simulink model "vnt_entire"  (R2018b)
settings: Solver=VariableStepAuto  StartTime=0.0  StopTime=inf  RelTol=1e-3
PreLoadFcn:
  | if exist('tl_preloadfcn','file'), tl_preloadfcn(gcs,'4.4.0.41'); end
PostLoadFcn:
  | if exist('tl_postloadfcn','file'), tl_postloadfcn(gcs,'4.4.0.41'); end
InitFcn:
  | if exist('tlds_init','file'), tlds_init(gcs); end
StartFcn:
  | if exist('tlds_start','file'), tlds_start(gcs); end
StopFcn:
  | if exist('tlds_stop','file'), tlds_stop(gcs); end
undefined symbols (not defined in the file): canChannel
libraries: canlib x29, canmsglib x27, simulink x4, pePwmGenerator x2, daqlib x1, aerolibnav x1
PreSaveFcn:
  | if exist('tl_presavefcn','file'), tl_presavefcn(gcs); end
CloseFcn:
  | if exist('tl_closefcn','file'), tl_closefcn(gcs); end
settings Model: Creator=GE72 6QF  LastModifiedBy=GE72 6QF

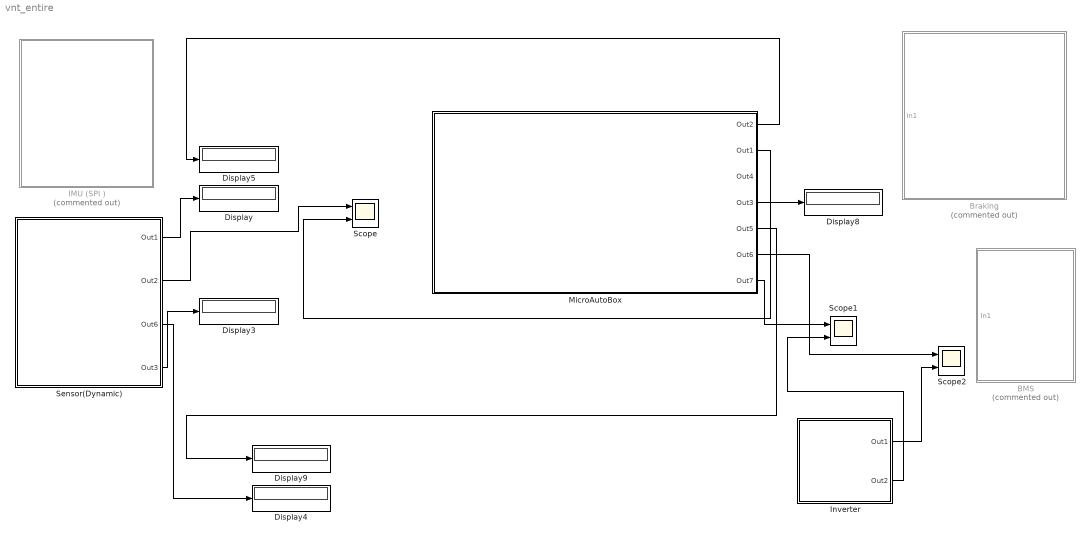
== system vnt_entire ==
  BMS : Subsystem  Commented=on
  Braking : Subsystem  Commented=on
  Display{,3..5,8..9} (6 alike) : Display
  IMU (SPI ) : Subsystem  Commented=on
  Inverter : Subsystem
  MicroAutoBox : Subsystem
  Scope : Scope  NumInputPorts=2
  Scope1 : Scope  NumInputPorts=2
  Scope2 : Scope  NumInputPorts=2
  Sensor(Dynamic) : Subsystem
  wires:
  Sensor(Dynamic)/1(Out1) -> Display/1
  Sensor(Dynamic)/3(Out6) -> Display4/1
  Inverter/2(Out2) -> Scope1/2
  MicroAutoBox/6(Out6) -> Scope2/1
  MicroAutoBox/7(Out7) -> Scope1/1
  MicroAutoBox/1(Out2) -> Display5/1
  MicroAutoBox/2(Out1) -> Scope/2
  MicroAutoBox/4(Out3) -> Display8/1
  MicroAutoBox/5(Out5) -> Display9/1
  Inverter/1(Out1) -> Scope2/2
  Sensor(Dynamic)/2(Out2) -> Scope/1
  Sensor(Dynamic)/4(Out3) -> Display3/1

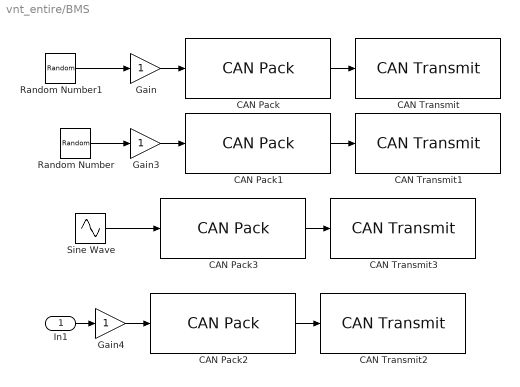
== system vnt_entire/BMS ==
  In1 : Inport
  CAN Pack : canmsglib/CAN Pack  MsgList=(none)  MsgName=CAN Msg  MsgIDType=Standard (11-bit identifier)  MsgIdentifier=100  MsgLength=8  SignalInfo=Signal1$0$8$1$1$1$0$1$0$-Inf$Inf$#  NSignals=1  StartBits=str2num('[int32(0)]')  SignalSizes=str2num('[int32(8)]')  ByteOrders=str2num('[int32(1)]')  DataTypes=str2num('[int32(1)]')  MultiplexTypes=str2num('[int32(1)]')  MultiplexValues=str2num('[double(0)]')  Factors=str2num('[double(1)]')  Offsets=str2num('[double(0)]')  Minimums=str2num('[double(-Inf)]')  Maximums=str2num('[double(Inf)]')  Remote=off  ApplyMinMax=off  BusOutput=off
      settings: SourceProductName=Simulink Real-Time  SourceProductBaseCode=XP  DataFormat=manually specified signals
  CAN Pack1 : canmsglib/CAN Pack  MsgList=(none)  MsgName=CAN Msg  MsgIDType=Standard (11-bit identifier)  MsgIdentifier=200  MsgLength=8  NSignals=0  StartBits=0  SignalSizes=0  ByteOrders=0  DataTypes=0  MultiplexTypes=0  MultiplexValues=0  Factors=0  Offsets=0  Minimums=0  Maximums=0  Remote=off  ApplyMinMax=off  BusOutput=off
      settings: SourceProductName=Simulink Real-Time  SourceProductBaseCode=XP  DataFormat=manually specified signals
  CAN Pack2 : canmsglib/CAN Pack  MsgList=(none)  MsgName=CAN Msg  MsgIDType=Standard (11-bit identifier)  MsgIdentifier=0  MsgLength=8  NSignals=0  StartBits=0  SignalSizes=0  ByteOrders=0  DataTypes=0  MultiplexTypes=0  MultiplexValues=0  Factors=0  Offsets=0  Minimums=0  Maximums=0  Remote=off  ApplyMinMax=off  BusOutput=off
      settings: SourceProductName=Simulink Real-Time  SourceProductBaseCode=XP  DataFormat=raw data
  CAN Pack3 : canmsglib/CAN Pack  MsgList=(none)  MsgName=CAN Msg  MsgIDType=Standard (11-bit identifier)  MsgIdentifier=0  MsgLength=8  NSignals=0  StartBits=0  SignalSizes=0  ByteOrders=0  DataTypes=0  MultiplexTypes=0  MultiplexValues=0  Factors=0  Offsets=0  Minimums=0  Maximums=0  Remote=off  ApplyMinMax=off  BusOutput=off
      settings: SourceProductName=Simulink Real-Time  SourceProductBaseCode=XP  DataFormat=raw data
  CAN Transmit : canlib/CAN Transmit  BlockHandle=11.0005  DeviceMenu=MathWorks Virtual 1 (Channel 1)  Device=MathWorks Virtual 1 (Channel 1)  ObjConstructor=canChannel('MathWorks', 'Virtual 1', 1)  EnablePeriodicTransmit=off  MessagePeriod=1.000
      settings: SourceProductName=Vehicle Network Toolbox  SourceProductBaseCode=VN
  CAN Transmit1 : canlib/CAN Transmit  BlockHandle=12.0005  DeviceMenu=MathWorks Virtual 1 (Channel 1)  Device=MathWorks Virtual 1 (Channel 1)  ObjConstructor=canChannel('MathWorks', 'Virtual 1', 1)  EnablePeriodicTransmit=off  MessagePeriod=1.000
      settings: SourceProductName=Vehicle Network Toolbox  SourceProductBaseCode=VN
  CAN Transmit2 : canlib/CAN Transmit  BlockHandle=13.0004  DeviceMenu=MathWorks Virtual 1 (Channel 1)  Device=MathWorks Virtual 1 (Channel 1)  ObjConstructor=canChannel('MathWorks', 'Virtual 1', 1)  EnablePeriodicTransmit=off  MessagePeriod=1.000
      settings: SourceProductName=Vehicle Network Toolbox  SourceProductBaseCode=VN
  CAN Transmit3 : canlib/CAN Transmit  BlockHandle=15.0005  DeviceMenu=MathWorks Virtual 1 (Channel 1)  Device=MathWorks Virtual 1 (Channel 1)  ObjConstructor=canChannel('MathWorks', 'Virtual 1', 1)  EnablePeriodicTransmit=off  MessagePeriod=1.000
      settings: SourceProductName=Vehicle Network Toolbox  SourceProductBaseCode=VN
  Gain : Gain
  Gain3 : Gain
  Gain4 : Gain
  Random Number : RandomNumber  SampleTime=0.1
  Random Number1 : RandomNumber  SampleTime=0.1
  Sine Wave : Sin  SampleTime=0
  wires:
  Gain4/1 -> CAN Pack2/1
  Random Number/1 -> Gain3/1
  CAN Pack3/1 -> CAN Transmit3/1
  Random Number1/1 -> Gain/1
  CAN Pack1/1 -> CAN Transmit1/1
  Gain3/1 -> CAN Pack1/1
  Gain/1 -> CAN Pack/1
  Sine Wave/1 -> CAN Pack3/1
  CAN Pack/1 -> CAN Transmit/1
  CAN Pack2/1 -> CAN Transmit2/1
  In1/1 -> Gain4/1

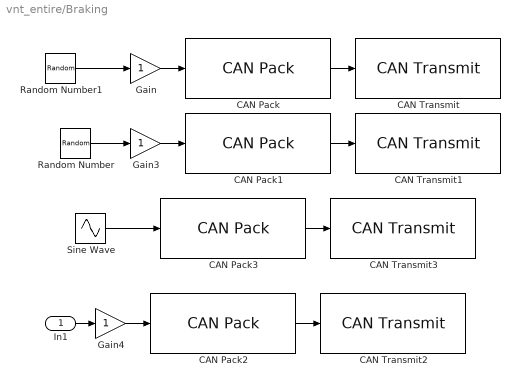
== system vnt_entire/Braking ==
  In1 : Inport
  CAN Pack : canmsglib/CAN Pack  MsgList=(none)  MsgName=CAN Msg  MsgIDType=Standard (11-bit identifier)  MsgIdentifier=100  MsgLength=8  SignalInfo=Signal1$0$8$1$1$1$0$1$0$-Inf$Inf$#  NSignals=1  StartBits=str2num('[int32(0)]')  SignalSizes=str2num('[int32(8)]')  ByteOrders=str2num('[int32(1)]')  DataTypes=str2num('[int32(1)]')  MultiplexTypes=str2num('[int32(1)]')  MultiplexValues=str2num('[double(0)]')  Factors=str2num('[double(1)]')  Offsets=str2num('[double(0)]')  Minimums=str2num('[double(-Inf)]')  Maximums=str2num('[double(Inf)]')  Remote=off  ApplyMinMax=off  BusOutput=off
      settings: SourceProductName=Simulink Real-Time  SourceProductBaseCode=XP  DataFormat=manually specified signals
  CAN Pack1 : canmsglib/CAN Pack  MsgList=(none)  MsgName=CAN Msg  MsgIDType=Standard (11-bit identifier)  MsgIdentifier=200  MsgLength=8  NSignals=0  StartBits=0  SignalSizes=0  ByteOrders=0  DataTypes=0  MultiplexTypes=0  MultiplexValues=0  Factors=0  Offsets=0  Minimums=0  Maximums=0  Remote=off  ApplyMinMax=off  BusOutput=off
      settings: SourceProductName=Simulink Real-Time  SourceProductBaseCode=XP  DataFormat=manually specified signals
  CAN Pack2 : canmsglib/CAN Pack  MsgList=(none)  MsgName=CAN Msg  MsgIDType=Standard (11-bit identifier)  MsgIdentifier=0  MsgLength=8  NSignals=0  StartBits=0  SignalSizes=0  ByteOrders=0  DataTypes=0  MultiplexTypes=0  MultiplexValues=0  Factors=0  Offsets=0  Minimums=0  Maximums=0  Remote=off  ApplyMinMax=off  BusOutput=off
      settings: SourceProductName=Simulink Real-Time  SourceProductBaseCode=XP  DataFormat=raw data
  CAN Pack3 : canmsglib/CAN Pack  MsgList=(none)  MsgName=CAN Msg  MsgIDType=Standard (11-bit identifier)  MsgIdentifier=0  MsgLength=8  NSignals=0  StartBits=0  SignalSizes=0  ByteOrders=0  DataTypes=0  MultiplexTypes=0  MultiplexValues=0  Factors=0  Offsets=0  Minimums=0  Maximums=0  Remote=off  ApplyMinMax=off  BusOutput=off
      settings: SourceProductName=Simulink Real-Time  SourceProductBaseCode=XP  DataFormat=raw data
  CAN Transmit : canlib/CAN Transmit  BlockHandle=46.0005  DeviceMenu=MathWorks Virtual 1 (Channel 1)  Device=MathWorks Virtual 1 (Channel 1)  ObjConstructor=canChannel('MathWorks', 'Virtual 1', 1)  EnablePeriodicTransmit=off  MessagePeriod=1.000
      settings: SourceProductName=Vehicle Network Toolbox  SourceProductBaseCode=VN
  CAN Transmit1 : canlib/CAN Transmit  BlockHandle=47.0005  DeviceMenu=MathWorks Virtual 1 (Channel 1)  Device=MathWorks Virtual 1 (Channel 1)  ObjConstructor=canChannel('MathWorks', 'Virtual 1', 1)  EnablePeriodicTransmit=off  MessagePeriod=1.000
      settings: SourceProductName=Vehicle Network Toolbox  SourceProductBaseCode=VN
  CAN Transmit2 : canlib/CAN Transmit  BlockHandle=48.0005  DeviceMenu=MathWorks Virtual 1 (Channel 1)  Device=MathWorks Virtual 1 (Channel 1)  ObjConstructor=canChannel('MathWorks', 'Virtual 1', 1)  EnablePeriodicTransmit=off  MessagePeriod=1.000
      settings: SourceProductName=Vehicle Network Toolbox  SourceProductBaseCode=VN
  CAN Transmit3 : canlib/CAN Transmit  BlockHandle=49.0005  DeviceMenu=MathWorks Virtual 1 (Channel 1)  Device=MathWorks Virtual 1 (Channel 1)  ObjConstructor=canChannel('MathWorks', 'Virtual 1', 1)  EnablePeriodicTransmit=off  MessagePeriod=1.000
      settings: SourceProductName=Vehicle Network Toolbox  SourceProductBaseCode=VN
  Gain : Gain
  Gain3 : Gain
  Gain4 : Gain
  Random Number : RandomNumber  SampleTime=0.1
  Random Number1 : RandomNumber  SampleTime=0.1
  Sine Wave : Sin  SampleTime=0
  wires:
  Gain4/1 -> CAN Pack2/1
  Random Number/1 -> Gain3/1
  CAN Pack3/1 -> CAN Transmit3/1
  Random Number1/1 -> Gain/1
  CAN Pack1/1 -> CAN Transmit1/1
  Gain3/1 -> CAN Pack1/1
  Gain/1 -> CAN Pack/1
  Sine Wave/1 -> CAN Pack3/1
  CAN Pack/1 -> CAN Transmit/1
  CAN Pack2/1 -> CAN Transmit2/1
  In1/1 -> Gain4/1

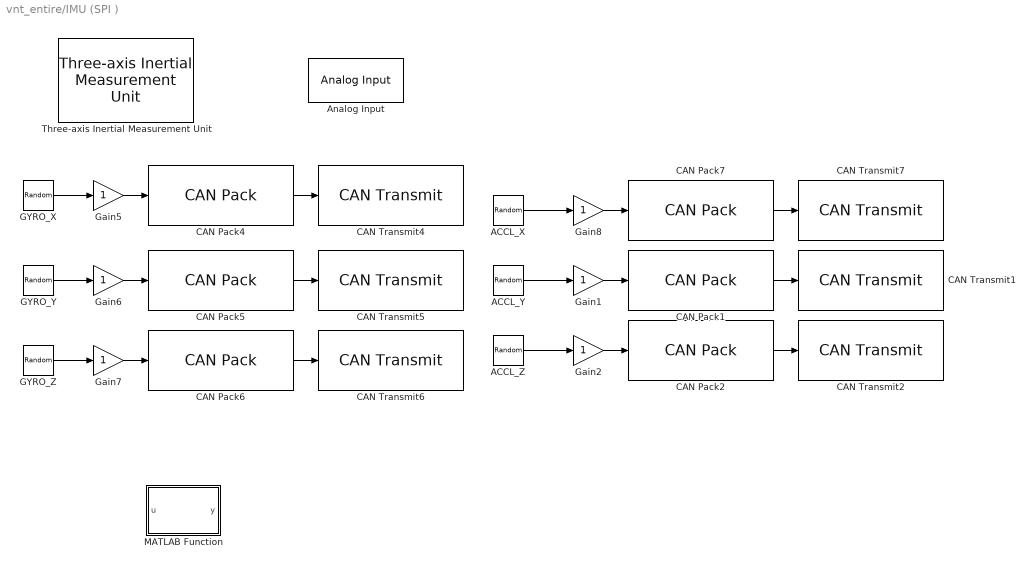
== system vnt_entire/IMU (SPI ) ==
  ACCL_X : RandomNumber  SampleTime=0.1
  ACCL_Y : RandomNumber  SampleTime=0.1
  ACCL_Z : RandomNumber  SampleTime=0.1
  Analog Input : daqlib/Analog Input  DeviceMenu=(none)  Device=(none)  NChannelsSelected=1  NPorts=1 for all channels  SampleRate=0  ActualRate=0  ScansPerTrigger=2  OutputTimestamp=off  AcqMode=0  NumFrameBuffer=100  OutputTriggertime=off
      settings: SourceProductName=Data Acquisition Toolbox  SourceProductBaseCode=DA
  CAN Pack{1..2,5..7} (5 alike) : canmsglib/CAN Pack  MsgList=(none)  MsgName=CAN Msg  MsgIDType=Standard (11-bit identifier)  MsgIdentifier=0  MsgLength=8  NSignals=0  StartBits=0  SignalSizes=0  ByteOrders=0  DataTypes=0  MultiplexTypes=0  MultiplexValues=0  Factors=0  Offsets=0  Minimums=0  Maximums=0  Remote=off  ApplyMinMax=off  BusOutput=off
      settings: SourceProductName=Simulink Real-Time  SourceProductBaseCode=XP  DataFormat=raw data
  CAN Pack4 : canmsglib/CAN Pack  MsgList=(none)  MsgName=CAN Msg  MsgIDType=Standard (11-bit identifier)  MsgIdentifier=150  MsgLength=8  SignalInfo=Signal1$0$8$1$1$1$0$1$0$-Inf$Inf$#  NSignals=1  StartBits=str2num('[int32(0)]')  SignalSizes=str2num('[int32(8)]')  ByteOrders=str2num('[int32(1)]')  DataTypes=str2num('[int32(1)]')  MultiplexTypes=str2num('[int32(1)]')  MultiplexValues=str2num('[double(0)]')  Factors=str2num('[double(1)]')  Offsets=str2num('[double(0)]')  Minimums=str2num('[double(-Inf)]')  Maximums=str2num('[double(Inf)]')  Remote=off  ApplyMinMax=off  BusOutput=off
      settings: SourceProductName=Simulink Real-Time  SourceProductBaseCode=XP  DataFormat=manually specified signals
  CAN Transmit1 : canlib/CAN Transmit  BlockHandle=84.001  DeviceMenu=MathWorks Virtual 1 (Channel 1)  Device=MathWorks Virtual 1 (Channel 1)  ObjConstructor=canChannel('MathWorks', 'Virtual 1', 1)  EnablePeriodicTransmit=off  MessagePeriod=1.000
      settings: SourceProductName=Vehicle Network Toolbox  SourceProductBaseCode=VN
  CAN Transmit2 : canlib/CAN Transmit  BlockHandle=85.0006  DeviceMenu=MathWorks Virtual 1 (Channel 1)  Device=MathWorks Virtual 1 (Channel 1)  ObjConstructor=canChannel('MathWorks', 'Virtual 1', 1)  EnablePeriodicTransmit=off  MessagePeriod=1.000
      settings: SourceProductName=Vehicle Network Toolbox  SourceProductBaseCode=VN
  CAN Transmit4 : canlib/CAN Transmit  BlockHandle=86.0006  DeviceMenu=MathWorks Virtual 1 (Channel 1)  Device=MathWorks Virtual 1 (Channel 1)  ObjConstructor=canChannel('MathWorks', 'Virtual 1', 1)  EnablePeriodicTransmit=off  MessagePeriod=1.000
      settings: SourceProductName=Vehicle Network Toolbox  SourceProductBaseCode=VN
  CAN Transmit5 : canlib/CAN Transmit  BlockHandle=87.0007  DeviceMenu=MathWorks Virtual 1 (Channel 1)  Device=MathWorks Virtual 1 (Channel 1)  ObjConstructor=canChannel('MathWorks', 'Virtual 1', 1)  EnablePeriodicTransmit=off  MessagePeriod=1.000
      settings: SourceProductName=Vehicle Network Toolbox  SourceProductBaseCode=VN
  CAN Transmit6 : canlib/CAN Transmit  BlockHandle=88.0007  DeviceMenu=MathWorks Virtual 1 (Channel 1)  Device=MathWorks Virtual 1 (Channel 1)  ObjConstructor=canChannel('MathWorks', 'Virtual 1', 1)  EnablePeriodicTransmit=off  MessagePeriod=1.000
      settings: SourceProductName=Vehicle Network Toolbox  SourceProductBaseCode=VN
  CAN Transmit7 : canlib/CAN Transmit  BlockHandle=89.0009  DeviceMenu=MathWorks Virtual 1 (Channel 1)  Device=MathWorks Virtual 1 (Channel 1)  ObjConstructor=canChannel('MathWorks', 'Virtual 1', 1)  EnablePeriodicTransmit=off  MessagePeriod=1.000
      settings: SourceProductName=Vehicle Network Toolbox  SourceProductBaseCode=VN
  GYRO_X : RandomNumber  SampleTime=0.1
  GYRO_Y : RandomNumber  SampleTime=0.1
  GYRO_Z : RandomNumber  SampleTime=0.1
  Gain{1..2,5..8} (6 alike) : Gain
  MATLAB Function : MATLAB Function  TreatAsAtomicUnit=on
  Three-axis Inertial Measurement Unit : aerolibnav/Three-axis Inertial Measurement Unit  units=Metric (MKS)  imu=[0 0 0]  i_Ts=0  dtype_a=on  w_a=190  z_a=0.707  a_sf_cc=[1 0 0; 0 1 0; 0 0 1]  a_bias=[0 0 0]  a_sat="[-inf  -inf  -inf  inf inf inf]"  dtype_g=on  w_g=190  z_g=0.707  g_sf_cc=[1 0 0; 0 1 0; 0 0 1]  g_bias=[0 0 0]  g_sens=[0 0 0]  g_sat="[-inf  -inf  -inf  inf inf inf]"  i_rand=on  i_seeds=[23093 23094 23095 23096 23097 23098]  i_pow=[0.001 0.001 0.001 0.0001 0.0001 0.0001]
  wires:
  Gain7/1 -> CAN Pack6/1
  CAN Pack5/1 -> CAN Transmit5/1
  Gain5/1 -> CAN Pack4/1
  CAN Pack4/1 -> CAN Transmit4/1
  Gain6/1 -> CAN Pack5/1
  Gain8/1 -> CAN Pack7/1
  CAN Pack7/1 -> CAN Transmit7/1
  CAN Pack6/1 -> CAN Transmit6/1
  ACCL_X/1 -> Gain8/1
  GYRO_X/1 -> Gain5/1
  GYRO_Z/1 -> Gain7/1
  GYRO_Y/1 -> Gain6/1
  Gain1/1 -> CAN Pack1/1
  CAN Pack1/1 -> CAN Transmit1/1
  ACCL_Y/1 -> Gain1/1
  Gain2/1 -> CAN Pack2/1
  CAN Pack2/1 -> CAN Transmit2/1
  ACCL_Z/1 -> Gain2/1

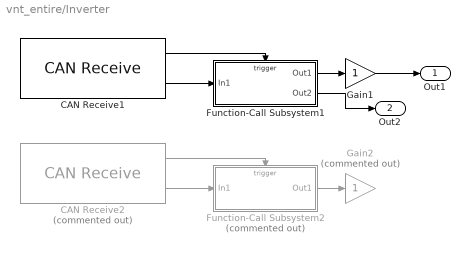
== system vnt_entire/Inverter ==
  CAN Receive1 : canlib/CAN Receive  BlockHandle=117.0006  DeviceMenu=MathWorks Virtual 1 (Channel 2)  Device=MathWorks Virtual 1 (Channel 2)  ObjConstructor=canChannel('MathWorks', 'Virtual 1', 2)  EnableStandardIDsFilter=off  StandardIDs=90  EnableExtendedIDsFilter=off  ExtendedIDs=0  SampleTime=0.01  MsgsPerTimestep=all  StdIDsCombo=Allow only  ExtIDsCombo=Allow all  InternalFilterUpdateStatus=on  BusOutput=off
      settings: SourceProductName=Vehicle Network Toolbox  SourceProductBaseCode=VN
  CAN Receive2 : canlib/CAN Receive  Commented=on  BlockHandle=118.0007  DeviceMenu=MathWorks Virtual 1 (Channel 2)  Device=MathWorks Virtual 1 (Channel 2)  ObjConstructor=canChannel('MathWorks', 'Virtual 1', 2)  EnableStandardIDsFilter=off  StandardIDs=90  EnableExtendedIDsFilter=off  ExtendedIDs=0  SampleTime=0.01  MsgsPerTimestep=all  StdIDsCombo=Allow only  ExtIDsCombo=Allow all  InternalFilterUpdateStatus=on  BusOutput=off
      settings: SourceProductName=Vehicle Network Toolbox  SourceProductBaseCode=VN
  Function-Call Subsystem1 : Subsystem  TreatAsAtomicUnit=on
  Function-Call Subsystem2 : Subsystem  Commented=on  TreatAsAtomicUnit=on
  Gain1 : Gain
  Gain2 : Gain  Commented=on
  Out1 : Outport
  Out2 : Outport  Port=2
  wires:
  Function-Call Subsystem2/1(Out1) -> Gain2/1
  CAN Receive1/1 -> Function-Call Subsystem1/Trigger
  Function-Call Subsystem1/1(Out1) -> Gain1/1
  CAN Receive2/2 -> Function-Call Subsystem2/1(In1)
  CAN Receive2/1 -> Function-Call Subsystem2/Trigger
  CAN Receive1/2 -> Function-Call Subsystem1/1(In1)
  Gain1/1 -> Out1/1
  Function-Call Subsystem1/2(Out2) -> Out2/1

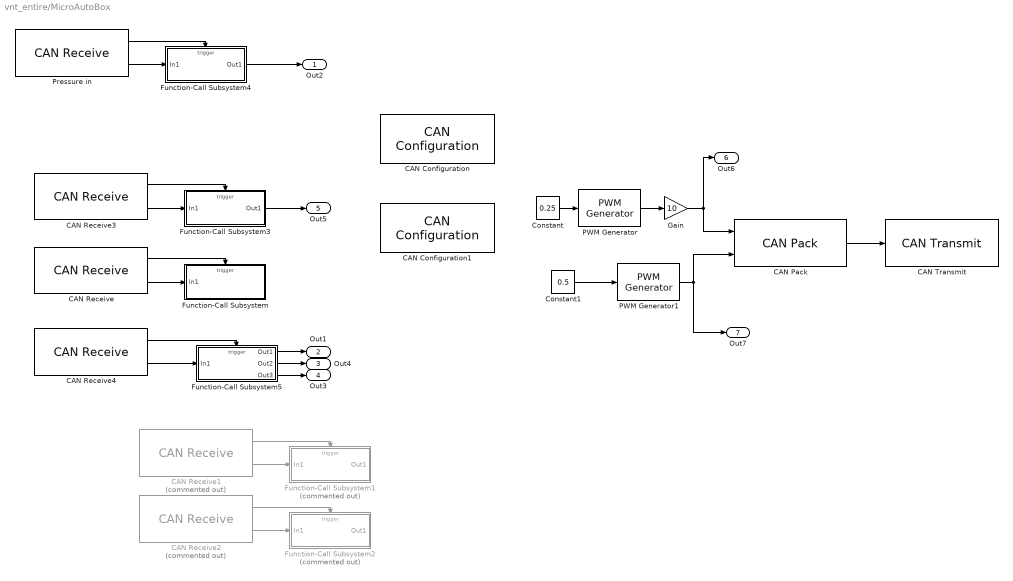
== system vnt_entire/MicroAutoBox ==
  CAN Configuration : canlib/CAN Configuration  BlockHandle=148.0005  DeviceMenu=MathWorks Virtual 1 (Channel 1)  Device=MathWorks Virtual 1 (Channel 1)  ObjConstructor=canChannel('MathWorks', 'Virtual 1', 1)  BusSpeed=500000  EnableBitParameters=off  AckMode=Normal
      settings: SourceProductName=Vehicle Network Toolbox  SourceProductBaseCode=VN
  CAN Configuration1 : canlib/CAN Configuration  BlockHandle=149.0005  DeviceMenu=MathWorks Virtual 1 (Channel 2)  Device=MathWorks Virtual 1 (Channel 2)  ObjConstructor=canChannel('MathWorks', 'Virtual 1', 2)  BusSpeed=500000  EnableBitParameters=off  AckMode=Normal
      settings: SourceProductName=Vehicle Network Toolbox  SourceProductBaseCode=VN
  CAN Pack : canmsglib/CAN Pack  MsgList=(none)  MsgName=CAN Msg  MsgIDType=Standard (11-bit identifier)  MsgIdentifier=90  MsgLength=8  SignalInfo=Signal1$0$32$1$3$1$0$1$0$-Inf$Inf$#Signal2$32$32$1$3$1$0$1$0$-Inf$Inf$#  NSignals=2  StartBits=str2num('[int32(0);int32(32)]')  SignalSizes=str2num('[int32(32);int32(32)]')  ByteOrders=str2num('[int32(1);int32(1)]')  DataTypes=str2num('[int32(3);int32(3)]')  MultiplexTypes=str2num('[int32(1);int32(1)]')  MultiplexValues=str2num('[double(0);double(0)]')  Factors=str2num('[double(1);double(1)]')  Offsets=str2num('[double(0);double(0)]')  Minimums=str2num('[double(-Inf);double(-Inf)]')  Maximums=str2num('[double(Inf);double(Inf)]')  Remote=off  ApplyMinMax=off  BusOutput=off
      settings: SourceProductName=Simulink Real-Time  SourceProductBaseCode=XP  DataFormat=manually specified signals
  CAN Receive : canlib/CAN Receive  BlockHandle=151.0006  DeviceMenu=MathWorks Virtual 1 (Channel 1)  Device=MathWorks Virtual 1 (Channel 1)  ObjConstructor=canChannel('MathWorks', 'Virtual 1', 1)  EnableStandardIDsFilter=off  StandardIDs=220  EnableExtendedIDsFilter=off  ExtendedIDs=0  SampleTime=0.01  MsgsPerTimestep=all  StdIDsCombo=Allow only  ExtIDsCombo=Allow all  InternalFilterUpdateStatus=on  BusOutput=off
      settings: SourceProductName=Vehicle Network Toolbox  SourceProductBaseCode=VN
  CAN Receive1 : canlib/CAN Receive  Commented=on  BlockHandle=152.0007  DeviceMenu=MathWorks Virtual 1 (Channel 1)  Device=MathWorks Virtual 1 (Channel 1)  ObjConstructor=canChannel('MathWorks', 'Virtual 1', 1)  EnableStandardIDsFilter=off  StandardIDs=0  EnableExtendedIDsFilter=off  ExtendedIDs=0  SampleTime=0.01  MsgsPerTimestep=all  StdIDsCombo=Allow all  ExtIDsCombo=Allow all  InternalFilterUpdateStatus=off  BusOutput=off
      settings: SourceProductName=Vehicle Network Toolbox  SourceProductBaseCode=VN
  CAN Receive2 : canlib/CAN Receive  Commented=on  BlockHandle=153.0006  DeviceMenu=MathWorks Virtual 1 (Channel 1)  Device=MathWorks Virtual 1 (Channel 1)  ObjConstructor=canChannel('MathWorks', 'Virtual 1', 1)  EnableStandardIDsFilter=off  StandardIDs=0  EnableExtendedIDsFilter=off  ExtendedIDs=0  SampleTime=0.01  MsgsPerTimestep=all  StdIDsCombo=Allow all  ExtIDsCombo=Allow all  InternalFilterUpdateStatus=off  BusOutput=off
      settings: SourceProductName=Vehicle Network Toolbox  SourceProductBaseCode=VN
  CAN Receive3 : canlib/CAN Receive  BlockHandle=154.0013  DeviceMenu=MathWorks Virtual 1 (Channel 2)  Device=MathWorks Virtual 1 (Channel 2)  ObjConstructor=canChannel('MathWorks', 'Virtual 1', 2)  EnableStandardIDsFilter=off  StandardIDs=230  EnableExtendedIDsFilter=off  ExtendedIDs=0  SampleTime=0.01  MsgsPerTimestep=all  StdIDsCombo=Allow only  ExtIDsCombo=Allow all  InternalFilterUpdateStatus=on  BusOutput=off
      settings: SourceProductName=Vehicle Network Toolbox  SourceProductBaseCode=VN
  CAN Receive4 : canlib/CAN Receive  BlockHandle=155.0007  DeviceMenu=MathWorks Virtual 1 (Channel 1)  Device=MathWorks Virtual 1 (Channel 1)  ObjConstructor=canChannel('MathWorks', 'Virtual 1', 1)  EnableStandardIDsFilter=off  StandardIDs=210  EnableExtendedIDsFilter=off  ExtendedIDs=0  SampleTime=0.01  MsgsPerTimestep=all  StdIDsCombo=Allow only  ExtIDsCombo=Allow all  InternalFilterUpdateStatus=on  BusOutput=off
      settings: SourceProductName=Vehicle Network Toolbox  SourceProductBaseCode=VN
  CAN Transmit : canlib/CAN Transmit  BlockHandle=156.0006  DeviceMenu=MathWorks Virtual 1 (Channel 2)  Device=MathWorks Virtual 1 (Channel 2)  ObjConstructor=canChannel('MathWorks', 'Virtual 1', 2)  EnablePeriodicTransmit=off  MessagePeriod=1.000
      settings: SourceProductName=Vehicle Network Toolbox  SourceProductBaseCode=VN
  Constant : Constant  Value=0.25
  Constant1 : Constant  Value=0.5
  Function-Call Subsystem : Subsystem  TreatAsAtomicUnit=on
  Function-Call Subsystem1 : Subsystem  Commented=on  TreatAsAtomicUnit=on
  Function-Call Subsystem2 : Subsystem  Commented=on  TreatAsAtomicUnit=on
  Function-Call Subsystem3 : Subsystem  TreatAsAtomicUnit=on
  Function-Call Subsystem4 : Subsystem  TreatAsAtomicUnit=on
  Function-Call Subsystem5 : Subsystem  TreatAsAtomicUnit=on
  Gain : Gain  Gain=10
  PWM Generator : pePwmGenerator/PWM Generator  CarrCount=Up  Tper=4  Ts=0.05
  PWM Generator1 : pePwmGenerator/PWM Generator  CarrCount=Up  Tper=4  Ts=0.05
  Pressure in : canlib/CAN Receive  BlockHandle=265.0013  DeviceMenu=MathWorks Virtual 1 (Channel 1)  Device=MathWorks Virtual 1 (Channel 1)  ObjConstructor=canChannel('MathWorks', 'Virtual 1', 1)  EnableStandardIDsFilter=off  StandardIDs=300  EnableExtendedIDsFilter=off  ExtendedIDs=0  SampleTime=0.01  MsgsPerTimestep=all  StdIDsCombo=Allow only  ExtIDsCombo=Allow all  InternalFilterUpdateStatus=on  BusOutput=off
      settings: SourceProductName=Vehicle Network Toolbox  SourceProductBaseCode=VN
  Out2 : Outport
  Out1 : Outport  Port=2
  Out4 : Outport  Port=3
  Out3 : Outport  Port=4
  Out5 : Outport  Port=5
  Out6 : Outport  Port=6
  Out7 : Outport  Port=7
  wires:
  CAN Receive/2 -> Function-Call Subsystem/1(In1)
  CAN Receive1/1 -> Function-Call Subsystem1/Trigger
  CAN Receive1/2 -> Function-Call Subsystem1/1(In1)
  CAN Receive2/1 -> Function-Call Subsystem2/Trigger
  CAN Receive2/2 -> Function-Call Subsystem2/1(In1)
  CAN Receive3/2 -> Function-Call Subsystem3/1(In1)
  Constant/1 -> PWM Generator/1
  CAN Pack/1 -> CAN Transmit/1
  PWM Generator/1 -> Gain/1
  Constant1/1 -> PWM Generator1/1
  Pressure in/2 -> Function-Call Subsystem4/1(In1)
  Function-Call Subsystem4/1(Out1) -> Out2/1
  CAN Receive4/2 -> Function-Call Subsystem5/1(In1)
  Function-Call Subsystem5/1(Out1) -> Out1/1
  Function-Call Subsystem5/2(Out2) -> Out4/1
  Function-Call Subsystem3/1(Out1) -> Out5/1
  Function-Call Subsystem5/3(Out3) -> Out3/1
  PWM Generator1/1 -> Out7/1, CAN Pack/2
  CAN Receive4/1 -> Function-Call Subsystem5/Trigger
  CAN Receive/1 -> Function-Call Subsystem/Trigger
  CAN Receive3/1 -> Function-Call Subsystem3/Trigger
  Pressure in/1 -> Function-Call Subsystem4/Trigger
  Gain/1 -> CAN Pack/1, Out6/1

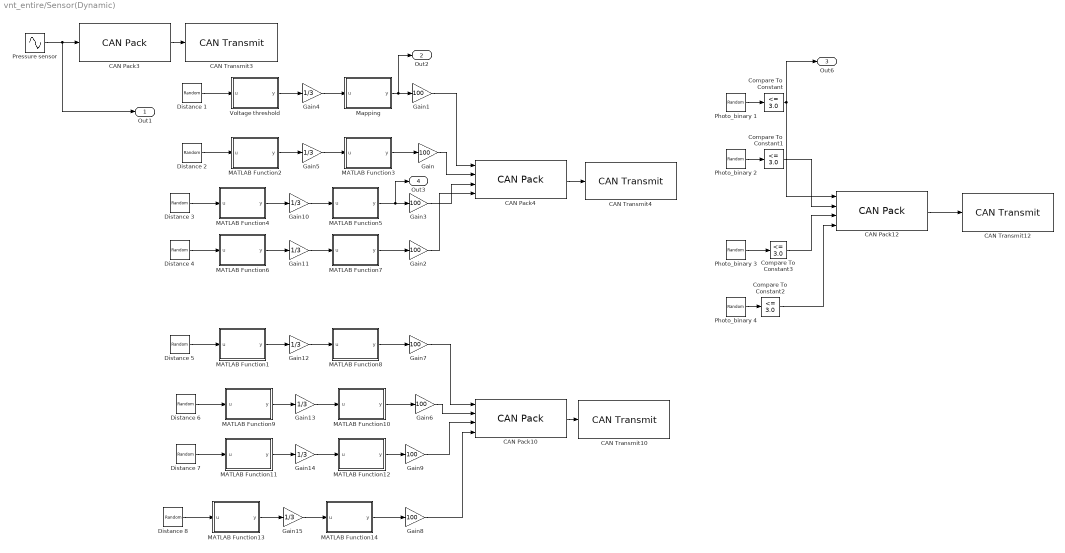
== system vnt_entire/Sensor(Dynamic) ==
  CAN Pack10 : canmsglib/CAN Pack  MsgList=(none)  MsgName=CAN Msg  MsgIDType=Standard (11-bit identifier)  MsgIdentifier=220  MsgLength=8  SignalInfo=Signal1$0$16$1$2$1$0$1$0$-Inf$Inf$#Signal2$16$16$1$2$1$0$1$0$-Inf$Inf$#Signal3$32$16$1$2$1$0$1$0$-Inf$Inf$#Signal4$48$16$1$2$1$0$1$0$-Inf$Inf$#  NSignals=4  StartBits=str2num('[int32(0);int32(16);int32(32);int32(48)]')  SignalSizes=str2num('[int32(16);int32(16);int32(16);int32(16)]')  ByteOrders=str2num('[int32(1);int32(1);int32(1);int32(1)]')  DataTypes=str2num('[int32(2);int32(2);int32(2);int32(2)]')  MultiplexTypes=str2num('[int32(1);int32(1);int32(1);int32(1)]')  MultiplexValues=str2num('[double(0);double(0);double(0);double(0)]')  Factors=str2num('[double(1);double(1);double(1);double(1)]')  Offsets=str2num('[double(0);double(0);double(0);double(0)]')  Minimums=str2num('[double(-Inf);double(-Inf);double(-Inf);double(-Inf)]')  Maximums=str2num('[double(Inf);double(Inf);double(Inf);double(Inf)]')  Remote=off  ApplyMinMax=off  BusOutput=off
      settings: SourceProductName=Simulink Real-Time  SourceProductBaseCode=XP  DataFormat=manually specified signals
  CAN Pack12 : canmsglib/CAN Pack  MsgList=(none)  MsgName=CAN Msg  MsgIDType=Standard (11-bit identifier)  MsgIdentifier=230  MsgLength=8  SignalInfo=Signal1$0$2$1$2$1$0$1$0$-Inf$Inf$#Signal2$2$2$1$2$1$0$1$0$-Inf$Inf$#Signal3$4$2$1$2$1$0$1$0$-Inf$Inf$#Signal4$6$2$1$2$1$0$1$0$-Inf$Inf$#  NSignals=4  StartBits=str2num('[int32(0);int32(2);int32(4);int32(6)]')  SignalSizes=str2num('[int32(2);int32(2);int32(2);int32(2)]')  ByteOrders=str2num('[int32(1);int32(1);int32(1);int32(1)]')  DataTypes=str2num('[int32(2);int32(2);int32(2);int32(2)]')  MultiplexTypes=str2num('[int32(1);int32(1);int32(1);int32(1)]')  MultiplexValues=str2num('[double(0);double(0);double(0);double(0)]')  Factors=str2num('[double(1);double(1);double(1);double(1)]')  Offsets=str2num('[double(0);double(0);double(0);double(0)]')  Minimums=str2num('[double(-Inf);double(-Inf);double(-Inf);double(-Inf)]')  Maximums=str2num('[double(Inf);double(Inf);double(Inf);double(Inf)]')  Remote=off  ApplyMinMax=off  BusOutput=off
      settings: SourceProductName=Simulink Real-Time  SourceProductBaseCode=XP  DataFormat=manually specified signals
  CAN Pack3 : canmsglib/CAN Pack  MsgList=(none)  MsgName=CAN Msg  MsgIDType=Standard (11-bit identifier)  MsgIdentifier=300  MsgLength=8  SignalInfo=Signal1$0$64$1$4$1$0$1$0$-Inf$Inf$#  NSignals=1  StartBits=str2num('[int32(0)]')  SignalSizes=str2num('[int32(64)]')  ByteOrders=str2num('[int32(1)]')  DataTypes=str2num('[int32(4)]')  MultiplexTypes=str2num('[int32(1)]')  MultiplexValues=str2num('[double(0)]')  Factors=str2num('[double(1)]')  Offsets=str2num('[double(0)]')  Minimums=str2num('[double(-Inf)]')  Maximums=str2num('[double(Inf)]')  Remote=off  ApplyMinMax=off  BusOutput=off
      settings: SourceProductName=Simulink Real-Time  SourceProductBaseCode=XP  DataFormat=manually specified signals
  CAN Pack4 : canmsglib/CAN Pack  MsgList=(none)  MsgName=CAN Msg  MsgIDType=Standard (11-bit identifier)  MsgIdentifier=210  MsgLength=8  SignalInfo=Signal1$0$16$1$2$1$0$1$0$-Inf$Inf$#Signal2$16$16$1$2$1$0$1$0$-Inf$Inf$#Signal3$32$16$1$2$1$0$1$0$-Inf$Inf$#Signal4$48$16$1$2$1$0$1$0$-Inf$Inf$#  NSignals=4  StartBits=str2num('[int32(0);int32(16);int32(32);int32(48)]')  SignalSizes=str2num('[int32(16);int32(16);int32(16);int32(16)]')  ByteOrders=str2num('[int32(1);int32(1);int32(1);int32(1)]')  DataTypes=str2num('[int32(2);int32(2);int32(2);int32(2)]')  MultiplexTypes=str2num('[int32(1);int32(1);int32(1);int32(1)]')  MultiplexValues=str2num('[double(0);double(0);double(0);double(0)]')  Factors=str2num('[double(1);double(1);double(1);double(1)]')  Offsets=str2num('[double(0);double(0);double(0);double(0)]')  Minimums=str2num('[double(-Inf);double(-Inf);double(-Inf);double(-Inf)]')  Maximums=str2num('[double(Inf);double(Inf);double(Inf);double(Inf)]')  Remote=off  ApplyMinMax=off  BusOutput=off
      settings: SourceProductName=Simulink Real-Time  SourceProductBaseCode=XP  DataFormat=manually specified signals
  CAN Transmit10 : canlib/CAN Transmit  BlockHandle=320.0005  DeviceMenu=MathWorks Virtual 1 (Channel 1)  Device=MathWorks Virtual 1 (Channel 1)  ObjConstructor=canChannel('MathWorks', 'Virtual 1', 1)  EnablePeriodicTransmit=off  MessagePeriod=1.000
      settings: SourceProductName=Vehicle Network Toolbox  SourceProductBaseCode=VN
  CAN Transmit12 : canlib/CAN Transmit  BlockHandle=321.0005  DeviceMenu=MathWorks Virtual 1 (Channel 1)  Device=MathWorks Virtual 1 (Channel 1)  ObjConstructor=canChannel('MathWorks', 'Virtual 1', 1)  EnablePeriodicTransmit=off  MessagePeriod=1.000
      settings: SourceProductName=Vehicle Network Toolbox  SourceProductBaseCode=VN
  CAN Transmit3 : canlib/CAN Transmit  BlockHandle=322.0005  DeviceMenu=MathWorks Virtual 1 (Channel 2)  Device=MathWorks Virtual 1 (Channel 2)  ObjConstructor=canChannel('MathWorks', 'Virtual 1', 2)  EnablePeriodicTransmit=off  MessagePeriod=1.000
      settings: SourceProductName=Vehicle Network Toolbox  SourceProductBaseCode=VN
  CAN Transmit4 : canlib/CAN Transmit  BlockHandle=323.0005  DeviceMenu=MathWorks Virtual 1 (Channel 1)  Device=MathWorks Virtual 1 (Channel 1)  ObjConstructor=canChannel('MathWorks', 'Virtual 1', 1)  EnablePeriodicTransmit=off  MessagePeriod=1.000
      settings: SourceProductName=Vehicle Network Toolbox  SourceProductBaseCode=VN
  Compare To Constant{,1..3} (4 alike) : simulink/Logic and Bit Operations/Compare To Constant  relop=<=  const=3.0  OutDataTypeStr=boolean
  Distance {1..8} (8 alike) : RandomNumber  Mean=5  Variance=5  SampleTime=0.1
  Gain{,1..3,6..9} (8 alike) : Gain  Gain=100
  Gain{4..5,10..15} (8 alike) : Gain  Gain=1/3
  MATLAB Function1 : MATLAB Function  TreatAsAtomicUnit=on
  MATLAB Function10 : MATLAB Function  TreatAsAtomicUnit=on
  MATLAB Function11 : MATLAB Function  TreatAsAtomicUnit=on
  MATLAB Function12 : MATLAB Function  TreatAsAtomicUnit=on
  MATLAB Function13 : MATLAB Function  TreatAsAtomicUnit=on
  MATLAB Function14 : MATLAB Function  TreatAsAtomicUnit=on
  MATLAB Function2 : MATLAB Function  TreatAsAtomicUnit=on
  MATLAB Function3 : MATLAB Function  TreatAsAtomicUnit=on
  MATLAB Function4 : MATLAB Function  TreatAsAtomicUnit=on
  MATLAB Function5 : MATLAB Function  TreatAsAtomicUnit=on
  MATLAB Function6 : MATLAB Function  TreatAsAtomicUnit=on
  MATLAB Function7 : MATLAB Function  TreatAsAtomicUnit=on
  MATLAB Function8 : MATLAB Function  TreatAsAtomicUnit=on
  MATLAB Function9 : MATLAB Function  TreatAsAtomicUnit=on
  "Mapping " : MATLAB Function  TreatAsAtomicUnit=on
  Photo_binary {1..4} (4 alike) : RandomNumber  Mean=3  SampleTime=0.1
  Pressure sensor : Sin  Amplitude=800  Bias=101300  SampleTime=0.001
  "Voltage threshold " : MATLAB Function  TreatAsAtomicUnit=on
  Out1 : Outport
  Out2 : Outport  Port=2
  Out6 : Outport  Port=3
  Out3 : Outport  Port=4
  wires:
  CAN Pack3/1 -> CAN Transmit3/1
  Gain3/1 -> CAN Pack4/3
  Gain/1 -> CAN Pack4/2
  Pressure sensor/1 -> Out1/1, CAN Pack3/1
  Gain1/1 -> CAN Pack4/1
  CAN Pack4/1 -> CAN Transmit4/1
  Gain2/1 -> CAN Pack4/4
  Photo_binary 1/1 -> Compare To Constant/1
  Gain6/1 -> CAN Pack10/2
  Gain9/1 -> CAN Pack10/3
  Compare To Constant3/1 -> CAN Pack12/3
  Gain7/1 -> CAN Pack10/1
  CAN Pack10/1 -> CAN Transmit10/1
  Photo_binary 3/1 -> Compare To Constant3/1
  Gain8/1 -> CAN Pack10/4
  CAN Pack12/1 -> CAN Transmit12/1
  Photo_binary 2/1 -> Compare To Constant1/1
  Compare To Constant1/1 -> CAN Pack12/2
  Photo_binary 4/1 -> Compare To Constant2/1
  Compare To Constant/1 -> CAN Pack12/1, Out6/1
  Compare To Constant2/1 -> CAN Pack12/4
  Distance 1/1 -> "Voltage threshold "/1(u)
  "Voltage threshold "/1(y) -> Gain4/1
  Gain4/1 -> "Mapping "/1(u)
  "Mapping "/1(y) -> Out2/1, Gain1/1
  Gain5/1 -> MATLAB Function3/1(u)
  Distance 2/1 -> MATLAB Function2/1(u)
  MATLAB Function3/1(y) -> Gain/1
  MATLAB Function2/1(y) -> Gain5/1
  MATLAB Function4/1(y) -> Gain10/1
  Gain10/1 -> MATLAB Function5/1(u)
  Distance 3/1 -> MATLAB Function4/1(u)
  MATLAB Function5/1(y) -> Out3/1, Gain3/1
  MATLAB Function6/1(y) -> Gain11/1
  Gain11/1 -> MATLAB Function7/1(u)
  Distance 4/1 -> MATLAB Function6/1(u)
  MATLAB Function7/1(y) -> Gain2/1
  Distance 5/1 -> MATLAB Function1/1(u)
  Gain12/1 -> MATLAB Function8/1(u)
  MATLAB Function1/1(y) -> Gain12/1
  MATLAB Function8/1(y) -> Gain7/1
  MATLAB Function10/1(y) -> Gain6/1
  Distance 6/1 -> MATLAB Function9/1(u)
  Gain13/1 -> MATLAB Function10/1(u)
  MATLAB Function9/1(y) -> Gain13/1
  MATLAB Function12/1(y) -> Gain9/1
  Distance 7/1 -> MATLAB Function11/1(u)
  Gain14/1 -> MATLAB Function12/1(u)
  MATLAB Function11/1(y) -> Gain14/1
  Distance 8/1 -> MATLAB Function13/1(u)
  Gain15/1 -> MATLAB Function14/1(u)
  MATLAB Function13/1(y) -> Gain15/1
  MATLAB Function14/1(y) -> Gain8/1

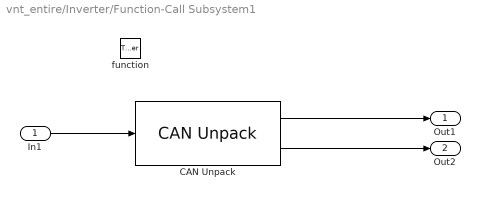
== system vnt_entire/Inverter/Function-Call Subsystem1 ==
  In1 : Inport
  function : TriggerPort  TriggerType=function-call  VariantControl=Variant
  CAN Unpack : canmsglib/CAN Unpack  MsgList=(none)  MsgName=CAN Msg  MsgIDType=Standard (11-bit identifier)  MsgIdentifier=90  MsgLength=8  SignalInfo=Signal1$0$32$1$3$1$0$1$0$-Inf$Inf$#Signal2$32$32$1$3$1$0$1$0$-Inf$Inf$#  NSignals=2  IDPort=off  TimestampPort=off  ErrorPort=off  RemotePort=off  LengthPort=off  StatusPort=off  StartBits=str2num('[int32(0);int32(32)]')  SignalSizes=str2num('[int32(32);int32(32)]')  ByteOrders=str2num('[int32(1);int32(1)]')  DataTypes=str2num('[int32(3);int32(3)]')  MultiplexTypes=str2num('[int32(1);int32(1)]')  MultiplexValues=str2num('[double(0);double(0)]')  Factors=str2num('[double(1);double(1)]')  Offsets=str2num('[double(0);double(0)]')  Minimums=str2num('[double(-Inf);double(-Inf)]')  Maximums=str2num('[double(Inf);double(Inf)]')  ApplyMinMax=off
      settings: SourceProductName=Simulink Real-Time  SourceProductBaseCode=XP
  Out1 : Outport
  Out2 : Outport  Port=2
  wires:
  In1/1 -> CAN Unpack/1
  CAN Unpack/1 -> Out1/1
  CAN Unpack/2 -> Out2/1

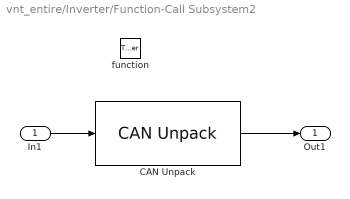
== system vnt_entire/Inverter/Function-Call Subsystem2 ==
  In1 : Inport
  function : TriggerPort  TriggerType=function-call  VariantControl=Variant
  CAN Unpack : canmsglib/CAN Unpack  MsgList=(none)  MsgName=CAN Msg  MsgIDType=Standard (11-bit identifier)  MsgIdentifier=90  MsgLength=8  SignalInfo=Signal1$0$8$1$1$1$0$1$0$-Inf$Inf$#  NSignals=1  IDPort=off  TimestampPort=off  ErrorPort=off  RemotePort=off  LengthPort=off  StatusPort=off  StartBits=str2num('[int32(0)]')  SignalSizes=str2num('[int32(8)]')  ByteOrders=str2num('[int32(1)]')  DataTypes=str2num('[int32(1)]')  MultiplexTypes=str2num('[int32(1)]')  MultiplexValues=str2num('[double(0)]')  Factors=str2num('[double(1)]')  Offsets=str2num('[double(0)]')  Minimums=str2num('[double(-Inf)]')  Maximums=str2num('[double(Inf)]')  ApplyMinMax=off
      settings: SourceProductName=Simulink Real-Time  SourceProductBaseCode=XP
  Out1 : Outport
  wires:
  In1/1 -> CAN Unpack/1
  CAN Unpack/1 -> Out1/1

== system vnt_entire/MicroAutoBox/Function-Call Subsystem ==
  In1 : Inport
  function : TriggerPort  TriggerType=function-call  VariantControl=Variant
  CAN Unpack : canmsglib/CAN Unpack  MsgList=(none)  MsgName=CAN Msg  MsgIDType=Standard (11-bit identifier)  MsgIdentifier=220  MsgLength=8  SignalInfo=Signal1$0$16$1$2$1$0$1$0$-Inf$Inf$#Signal2$16$16$1$2$1$0$1$0$-Inf$Inf$#Signal3$32$16$1$2$1$0$1$0$-Inf$Inf$#Signal4$48$16$1$2$1$0$1$0$-Inf$Inf$#  NSignals=4  IDPort=off  TimestampPort=off  ErrorPort=off  RemotePort=off  LengthPort=off  StatusPort=off  StartBits=str2num('[int32(0);int32(16);int32(32);int32(48)]')  SignalSizes=str2num('[int32(16);int32(16);int32(16);int32(16)]')  ByteOrders=str2num('[int32(1);int32(1);int32(1);int32(1)]')  DataTypes=str2num('[int32(2);int32(2);int32(2);int32(2)]')  MultiplexTypes=str2num('[int32(1);int32(1);int32(1);int32(1)]')  MultiplexValues=str2num('[double(0);double(0);double(0);double(0)]')  Factors=str2num('[double(1);double(1);double(1);double(1)]')  Offsets=str2num('[double(0);double(0);double(0);double(0)]')  Minimums=str2num('[double(-Inf);double(-Inf);double(-Inf);double(-Inf)]')  Maximums=str2num('[double(Inf);double(Inf);double(Inf);double(Inf)]')  ApplyMinMax=off
      settings: SourceProductName=Simulink Real-Time  SourceProductBaseCode=XP
  wires:
  In1/1 -> CAN Unpack/1

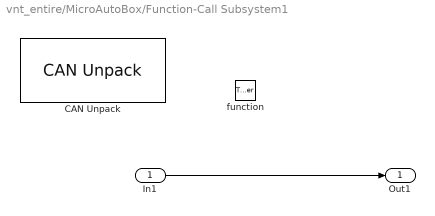
== system vnt_entire/MicroAutoBox/Function-Call Subsystem1 ==
  In1 : Inport
  function : TriggerPort  TriggerType=function-call  VariantControl=Variant
  CAN Unpack : canmsglib/CAN Unpack  MsgName=CAN Msg  MsgIDType=Standard (11-bit identifier)  MsgIdentifier=0  MsgLength=8  NSignals=0  IDPort=off  TimestampPort=off  ErrorPort=off  RemotePort=off  LengthPort=off  StatusPort=off  StartBits=0  SignalSizes=0  ByteOrders=0  DataTypes=0  MultiplexTypes=0  MultiplexValues=0  Factors=0  Offsets=0  Minimums=0  Maximums=0  ApplyMinMax=off
      settings: SourceProductName=Simulink Real-Time  SourceProductBaseCode=XP  DataFormat=raw data
  Out1 : Outport
  wires:
  In1/1 -> Out1/1

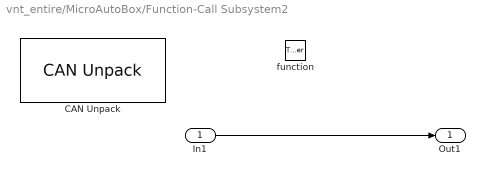
== system vnt_entire/MicroAutoBox/Function-Call Subsystem2 ==
  In1 : Inport
  function : TriggerPort  TriggerType=function-call  VariantControl=Variant
  CAN Unpack : canmsglib/CAN Unpack  MsgName=CAN Msg  MsgIDType=Standard (11-bit identifier)  MsgIdentifier=0  MsgLength=8  NSignals=0  IDPort=off  TimestampPort=off  ErrorPort=off  RemotePort=off  LengthPort=off  StatusPort=off  StartBits=0  SignalSizes=0  ByteOrders=0  DataTypes=0  MultiplexTypes=0  MultiplexValues=0  Factors=0  Offsets=0  Minimums=0  Maximums=0  ApplyMinMax=off
      settings: SourceProductName=Simulink Real-Time  SourceProductBaseCode=XP  DataFormat=raw data
  Out1 : Outport
  wires:
  In1/1 -> Out1/1

== system vnt_entire/MicroAutoBox/Function-Call Subsystem3 ==
  In1 : Inport
  function : TriggerPort  TriggerType=function-call  VariantControl=Variant
  CAN Unpack : canmsglib/CAN Unpack  MsgList=(none)  MsgName=CAN Msg  MsgIDType=Standard (11-bit identifier)  MsgIdentifier=230  MsgLength=8  SignalInfo=Signal1$0$2$1$2$1$0$1$0$-Inf$Inf$#Signal2$2$2$1$2$1$0$1$0$-Inf$Inf$#Signal3$4$2$1$2$1$0$1$0$-Inf$Inf$#Signal4$6$2$1$2$1$0$1$0$-Inf$Inf$#  NSignals=4  IDPort=off  TimestampPort=off  ErrorPort=off  RemotePort=off  LengthPort=off  StatusPort=off  StartBits=str2num('[int32(0);int32(2);int32(4);int32(6)]')  SignalSizes=str2num('[int32(2);int32(2);int32(2);int32(2)]')  ByteOrders=str2num('[int32(1);int32(1);int32(1);int32(1)]')  DataTypes=str2num('[int32(2);int32(2);int32(2);int32(2)]')  MultiplexTypes=str2num('[int32(1);int32(1);int32(1);int32(1)]')  MultiplexValues=str2num('[double(0);double(0);double(0);double(0)]')  Factors=str2num('[double(1);double(1);double(1);double(1)]')  Offsets=str2num('[double(0);double(0);double(0);double(0)]')  Minimums=str2num('[double(-Inf);double(-Inf);double(-Inf);double(-Inf)]')  Maximums=str2num('[double(Inf);double(Inf);double(Inf);double(Inf)]')  ApplyMinMax=off
      settings: SourceProductName=Simulink Real-Time  SourceProductBaseCode=XP
  Out1 : Outport
  wires:
  In1/1 -> CAN Unpack/1
  CAN Unpack/1 -> Out1/1

== system vnt_entire/MicroAutoBox/Function-Call Subsystem4 ==
  In1 : Inport
  function : TriggerPort  TriggerType=function-call  VariantControl=Variant
  CAN Unpack : canmsglib/CAN Unpack  MsgList=(none)  MsgName=CAN Msg  MsgIDType=Standard (11-bit identifier)  MsgIdentifier=300  MsgLength=8  SignalInfo=Signal1$0$64$1$4$1$0$1$0$-Inf$Inf$#  NSignals=1  IDPort=off  TimestampPort=off  ErrorPort=off  RemotePort=off  LengthPort=off  StatusPort=off  StartBits=str2num('[int32(0)]')  SignalSizes=str2num('[int32(64)]')  ByteOrders=str2num('[int32(1)]')  DataTypes=str2num('[int32(4)]')  MultiplexTypes=str2num('[int32(1)]')  MultiplexValues=str2num('[double(0)]')  Factors=str2num('[double(1)]')  Offsets=str2num('[double(0)]')  Minimums=str2num('[double(-Inf)]')  Maximums=str2num('[double(Inf)]')  ApplyMinMax=off
      settings: SourceProductName=Simulink Real-Time  SourceProductBaseCode=XP
  Out1 : Outport
  wires:
  In1/1 -> CAN Unpack/1
  CAN Unpack/1 -> Out1/1

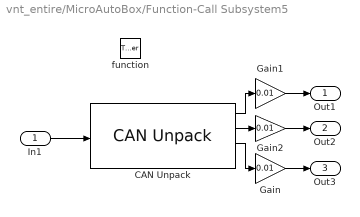
== system vnt_entire/MicroAutoBox/Function-Call Subsystem5 ==
  In1 : Inport
  function : TriggerPort  TriggerType=function-call  VariantControl=Variant
  CAN Unpack : canmsglib/CAN Unpack  MsgList=(none)  MsgName=CAN Msg  MsgIDType=Standard (11-bit identifier)  MsgIdentifier=210  MsgLength=8  SignalInfo=Signal1$0$16$1$2$1$0$1$0$-Inf$Inf$#Signal2$16$16$1$2$1$0$1$0$-Inf$Inf$#Signal3$32$16$1$2$1$0$1$0$-Inf$Inf$#Signal4$48$16$1$2$1$0$1$0$-Inf$Inf$#  NSignals=4  IDPort=off  TimestampPort=off  ErrorPort=off  RemotePort=off  LengthPort=off  StatusPort=off  StartBits=str2num('[int32(0);int32(16);int32(32);int32(48)]')  SignalSizes=str2num('[int32(16);int32(16);int32(16);int32(16)]')  ByteOrders=str2num('[int32(1);int32(1);int32(1);int32(1)]')  DataTypes=str2num('[int32(2);int32(2);int32(2);int32(2)]')  MultiplexTypes=str2num('[int32(1);int32(1);int32(1);int32(1)]')  MultiplexValues=str2num('[double(0);double(0);double(0);double(0)]')  Factors=str2num('[double(1);double(1);double(1);double(1)]')  Offsets=str2num('[double(0);double(0);double(0);double(0)]')  Minimums=str2num('[double(-Inf);double(-Inf);double(-Inf);double(-Inf)]')  Maximums=str2num('[double(Inf);double(Inf);double(Inf);double(Inf)]')  ApplyMinMax=off
      settings: SourceProductName=Simulink Real-Time  SourceProductBaseCode=XP
  Gain : Gain  Gain=0.01
  Gain1 : Gain  Gain=0.01
  Gain2 : Gain  Gain=0.01
  Out1 : Outport
  Out2 : Outport  Port=2
  Out3 : Outport  Port=3
  wires:
  In1/1 -> CAN Unpack/1
  CAN Unpack/1 -> Gain1/1
  Gain1/1 -> Out1/1
  CAN Unpack/2 -> Gain2/1
  Gain2/1 -> Out2/1
  CAN Unpack/3 -> Gain/1
  Gain/1 -> Out3/1

== matlab function vnt_entire/Sensor(Dynamic)/Mapping  ==
  data: u input; y output
function y = fcn(u)
    % 0 to 1023 -> 2mm to 8 mm
    y = mappp(u, 0, 3.333, 2, 8);
end
function res = mappp(voltage, from1, from2, to1, to2)
    res = to1 + (voltage-from1)*(to2-to1)/(from2-from1);
end

== matlab function vnt_entire/Sensor(Dynamic)/Voltage threshold  ==
  data: u input; y output
function y = fcn(u)
if u >= 0 && u <= 10 
    y= u;
else
    y = 0;
end
end

== matlab function vnt_entire/Sensor(Dynamic)/MATLAB Function2 ==
  data: u input; y output
function y = fcn(u)
if u >= 0 && u <= 10 
    y= u;
else
    y = 0;
end
end

== matlab function vnt_entire/Sensor(Dynamic)/MATLAB Function3 ==
  data: u input; y output
function y = fcn(u)
    % 0 to 1023 -> 2mm to 8 mm
    y = mappp(u, 0, 3.333, 2, 8);
end
function res = mappp(voltage, from1, from2, to1, to2)
    res = to1 + (voltage-from1)*(to2-to1)/(from2-from1);
end

== matlab function vnt_entire/Sensor(Dynamic)/MATLAB Function4 ==
  data: u input; y output
function y = fcn(u)
if u >= 0 && u <= 10 
    y= u;
else
    y = 0;
end
end

== matlab function vnt_entire/Sensor(Dynamic)/MATLAB Function5 ==
  data: u input; y output
function y = fcn(u)
    % 0 to 1023 -> 2mm to 8 mm
    y = mappp(u, 0, 3.333, 2, 8);
end
function res = mappp(voltage, from1, from2, to1, to2)
    res = to1 + (voltage-from1)*(to2-to1)/(from2-from1);
end

== matlab function vnt_entire/Sensor(Dynamic)/MATLAB Function6 ==
  data: u input; y output
function y = fcn(u)
if u >= 0 && u <= 10 
    y= u;
else
    y = 0;
end
end

== matlab function vnt_entire/Sensor(Dynamic)/MATLAB Function7 ==
  data: u input; y output
function y = fcn(u)
    % 0 to 1023 -> 2mm to 8 mm
    y = mappp(u, 0, 3.333, 2, 8);
end
function res = mappp(voltage, from1, from2, to1, to2)
    res = to1 + (voltage-from1)*(to2-to1)/(from2-from1);
end

== matlab function vnt_entire/Sensor(Dynamic)/MATLAB Function1 ==
  data: u input; y output
function y = fcn(u)
if u >= 0 && u <= 10 
    y= u;
else
    y = 0;
end
end

== matlab function vnt_entire/Sensor(Dynamic)/MATLAB Function8 ==
  data: u input; y output
function y = fcn(u)
    % 0 to 1023 -> 2mm to 8 mm
    y = mappp(u, 0, 3.333, 2, 8);
end
function res = mappp(voltage, from1, from2, to1, to2)
    res = to1 + (voltage-from1)*(to2-to1)/(from2-from1);
end

== matlab function vnt_entire/Sensor(Dynamic)/MATLAB Function10 ==
  data: u input; y output
function y = fcn(u)
    % 0 to 1023 -> 2mm to 8 mm
    y = mappp(u, 0, 3.333, 2, 8);
end
function res = mappp(voltage, from1, from2, to1, to2)
    res = to1 + (voltage-from1)*(to2-to1)/(from2-from1);
end

== matlab function vnt_entire/Sensor(Dynamic)/MATLAB Function9 ==
  data: u input; y output
function y = fcn(u)
if u >= 0 && u <= 10 
    y= u;
else
    y = 0;
end
end

== matlab function vnt_entire/Sensor(Dynamic)/MATLAB Function11 ==
  data: u input; y output
function y = fcn(u)
if u >= 0 && u <= 10 
    y= u;
else
    y = 0;
end
end

== matlab function vnt_entire/Sensor(Dynamic)/MATLAB Function12 ==
  data: u input; y output
function y = fcn(u)
    % 0 to 1023 -> 2mm to 8 mm
    y = mappp(u, 0, 3.333, 2, 8);
end
function res = mappp(voltage, from1, from2, to1, to2)
    res = to1 + (voltage-from1)*(to2-to1)/(from2-from1);
end

== matlab function vnt_entire/Sensor(Dynamic)/MATLAB Function13 ==
  data: u input; y output
function y = fcn(u)
if u >= 0 && u <= 10 
    y= u;
else
    y = 0;
end
end

== matlab function vnt_entire/Sensor(Dynamic)/MATLAB Function14 ==
  data: u input; y output
function y = fcn(u)
    % 0 to 1023 -> 2mm to 8 mm
    y = mappp(u, 0, 3.333, 2, 8);
end
function res = mappp(voltage, from1, from2, to1, to2)
    res = to1 + (voltage-from1)*(to2-to1)/(from2-from1);
end

== matlab function vnt_entire/IMU (SPI )/MATLAB Function ==
  data: u input; y output
function y = fcn(u)

y = u;
